simulink model "alpha_en_fct_couple"  (R2024b)
settings: Solver=VariableStepAuto  StartTime=0.0  StopTime=30  RelTol=1e-3
values from neighbouring files (symbols this model uses):
  alpha_d_ini = 0    [projet.m]
  alpha_g_ini = 0    [projet.m]
  dalpha_d_ini = 0    [projet.m]
  dalpha_g_ini = 0    [projet.m]
libraries: simulink x2
settings Model: Creator=yann  LastModifiedBy=yann

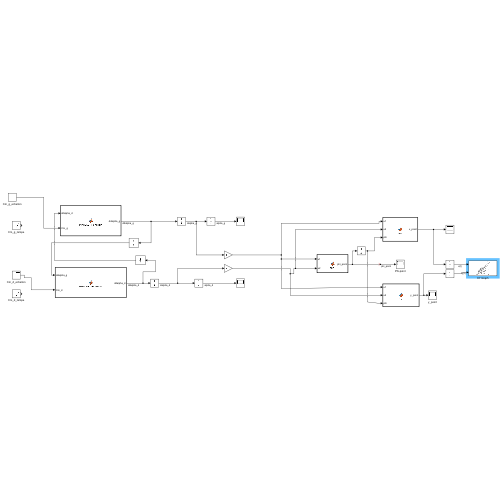
[thumbnail: Simulink's stored preview of the top-level diagram]
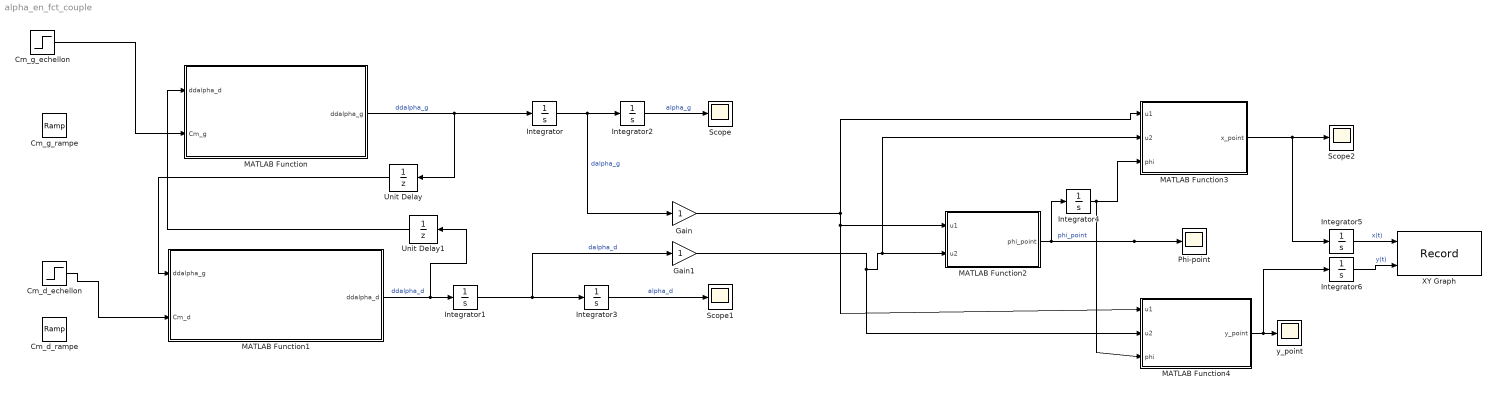
== system alpha_en_fct_couple ==
  Cm_d_echellon : Step  After=0  SampleTime=0
  Cm_d_rampe : simulink/Sources/Ramp  slope=1  start=0  InitialOutput=0
  Cm_g_echellon : Step  After=0  SampleTime=0
  Cm_g_rampe : simulink/Sources/Ramp  slope=1  start=0  InitialOutput=0
  Gain : Gain
  Gain1 : Gain
  Integrator : Integrator  InitialCondition=dalpha_g_ini
  Integrator1 : Integrator  InitialCondition=dalpha_d_ini
  Integrator2 : Integrator  InitialCondition=alpha_g_ini
  Integrator3 : Integrator  InitialCondition=alpha_d_ini
  Integrator4 : Integrator
  Integrator5 : Integrator
  Integrator6 : Integrator
  MATLAB Function : MATLAB Function  TreatAsAtomicUnit=on
  MATLAB Function1 : MATLAB Function  TreatAsAtomicUnit=on
  MATLAB Function2 : MATLAB Function  TreatAsAtomicUnit=on
  MATLAB Function3 : MATLAB Function  TreatAsAtomicUnit=on
  MATLAB Function4 : MATLAB Function  TreatAsAtomicUnit=on
  Phi-point : Scope
  Scope : Scope
  Scope1 : Scope
  Scope2 : Scope
  Unit Delay : UnitDelay  SampleTime=-1  HasFrameUpgradeWarning=on
  Unit Delay1 : UnitDelay  SampleTime=-1  HasFrameUpgradeWarning=on
  XY Graph : Record  FileSettingsInternal="{\"entries\":[{\"content\":{\"excelSettings\":{\"content\":{},\"type\":\"Streamout.ExcelSettings\"}},\"type\":\"Streamout.FileSettingStorage\",\"uuid\":\"\"}],\"packageUris\":[\"http:\\/\\/schema.mathworks.com\\/mf0\\/streamout_blocks\\/R2020a\"],\"version\":\"1.0\"}"  Layout=[1 1]  SignalsInternal="{\"entries\":[{\"content\":{\"signals\":[{\"content\":{\"blockPath\":[],\"dimensions\":[1],\"domain\":\"\",\"lineColor\":\"#a2142f\",\"plots\":[ 1 ],\"port\":1,\"sid\":[\"\"],\"signalID\":1,\"signalName\":\"x(t)\"},\"type\":\"RecordBlkView.Signal\",\"uuid\":\"\"},{\"content\":{\"blockPath\":[],\"dimensions\":[1],\"domain\":\"\",\"lineColor\":\"#139fff\",\"plots\":[ 1 ],\"port\":2,\"sid\":[\"\"],\"signalID\":2,\"signalName\":\"y(t)\"},\"type\":\"RecordBlkView.Signal\",\"uuid\":\"\"}]},\"type\":\"RecordBlkView.InputSignals\",\"uuid\":\"\"}],\"packageUris\":[\"http:\\/\\/schema.mathworks.com\\/mf0\\/streamout_blocks\\/R2020a\"],\"version\":\"1.0\"}"  VisualizationBindings="{\"xyplotplugin\":{\"info\":[{\"series\":[{\"bindingParametersList\":[{\"parameter\":\"X-Axis\",\"signalID\":1,\"signalName\":\"x(t)\"},{\"parameter\":\"Y-Axis\",\"signalID\":2,\"signalName\":\"y(t)\"}],\"seriesID\":0}],\"subplotID\":1}]}}"  CompatibilityTag=XY
  y_point : Scope
  wires:
  MATLAB Function/1(ddalpha_g) -> Unit Delay/1, Integrator/1  "ddalpha_g"
  Integrator/1 -> Gain/1, Integrator2/1  "dalpha_g"
  MATLAB Function1/1(ddalpha_d) -> Unit Delay1/1, Integrator1/1  "ddalpha_d"
  Integrator1/1 -> Gain1/1, Integrator3/1  "dalpha_d"
  Integrator2/1 -> Scope/1  "alpha_g"
  Integrator3/1 -> Scope1/1  "alpha_d"
  Cm_g_echellon/1 -> MATLAB Function/2(Cm_g)
  Cm_d_echellon/1 -> MATLAB Function1/2(Cm_d)
  Unit Delay1/1 -> MATLAB Function/1(ddalpha_d)
  Unit Delay/1 -> MATLAB Function1/1(ddalpha_g)
  Integrator5/1 -> XY Graph/1  "x(t)"
  MATLAB Function2/1(phi_point) -> Phi-point/1, Integrator4/1  "phi_point"
  Gain1/1 -> MATLAB Function4/2(u2), MATLAB Function3/2(u2), MATLAB Function2/2(u2)
  Gain/1 -> MATLAB Function4/1(u1), MATLAB Function2/1(u1), MATLAB Function3/1(u1)
  MATLAB Function4/1(y_point) -> Integrator6/1, y_point/1
  MATLAB Function3/1(x_point) -> Integrator5/1, Scope2/1
  Integrator6/1 -> XY Graph/2  "y(t)"
  Integrator4/1 -> MATLAB Function3/3(phi), MATLAB Function4/3(phi)

== matlab function alpha_en_fct_couple/MATLAB Function ==
  data: ddalpha_d input; ddalpha_g output; Cm_g input
function ddalpha_g = MATLAB_Function(ddalpha_d,Cm_g)
h=2;
l=15e-2;
L=2*l;
R=10e-2;
m_B=750;
e=2e-2;
rho=1200;
mr=300e-3;
I = m_B * (L*2 + h*2) / 12;
Ie = rho*R^2;
I_orth =1/4*mr*R*2+1/10*mr*e*2;


ddalpha_g = (-2*(0.5*I + I_orth)*(R^2/(8*l^2))*ddalpha_d+Cm_g);
ddalpha_g=ddalpha_g/(2*(0.5*I+I_orth)*(R^2/(8*l^2))-Ie+0.5*m_B*R^2);

== matlab function alpha_en_fct_couple/MATLAB Function2 ==
  data: u1 input; phi_point output; u2 input
function phi_point = fcn(u1, u2)
    

    phi_point = (-10 /30) *(u1+u2); 
end

== matlab function alpha_en_fct_couple/MATLAB Function1 ==
  data: ddalpha_g input; ddalpha_d output; Cm_d input
function ddalpha_d = MATLAB_Function(ddalpha_g,Cm_d)
h=2;
l=15e-2;
R=10e-2;
m_B=750;
e=2e-2;
L=2*l;
rho=1200;
mr=300e-3;
I = m_B * (L*2 + h*2) / 12;
Ie = rho*R^2;
I_orth =1/4*mr*R*2+1/10*mr*e*2;


ddalpha_d = (-2*(0.5*I + I_orth)*(R^2/(8*l^2))*ddalpha_g+Cm_d);
ddalpha_d=ddalpha_d/(2*(0.5*I+I_orth)*(R^2/(8*l^2))+Ie+0.5*m_B*R^2);

== matlab function alpha_en_fct_couple/MATLAB Function3 ==
  data: u1 input; x_point output; u2 input; phi input
function x_point = fcn(u1,u2,phi)
    x_point = (10/2)*((u1+u2)*cos(phi)+(u2-u1)*sin(phi));
end

== matlab function alpha_en_fct_couple/MATLAB Function4 ==
  data: u1 input; y_point output; u2 input; phi input
function y_point = fcn(u1,u2,phi)
    y_point = (10/2)*((u1-u2)*cos(phi)+(u2+u1)*sin(phi));
end
